simulink model "pwm"  (R2015b)
settings: Solver=ode4  StartTime=0.0  StopTime=10  FixedStep=0.1  RelTol=1e-3
libraries: simulink x2
settings Model: Creator=sat_lab  LastModifiedBy=sat_lab

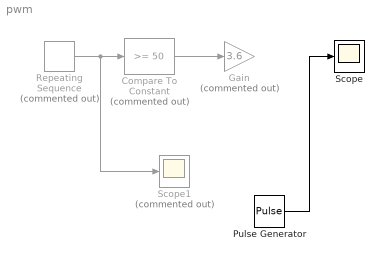
== system pwm ==
  Compare To Constant : simulink/Logic and Bit Operations/Compare To Constant  Commented=on  relop=>=  const=50  OutDataTypeStr=boolean
  Gain : Gain  Commented=on  Gain=3.6
  Pulse Generator : DiscretePulseGenerator  PulseType=Time based  Period=0.001  PulseWidth=5
  Repeating Sequence : simulink/Sources/Repeating Sequence  Commented=on  rep_seq_t=[0 0.2]  rep_seq_y=[0 100]
  Scope : Scope
  Scope1 : Scope  Commented=on
  wires:
  Repeating Sequence/1 -> Scope1/1, Compare To Constant/1
  Compare To Constant/1 -> Gain/1
  Pulse Generator/1 -> Scope/1
